simulink model "unicycle_control"  (R2015a)
settings: Solver=ode45  StartTime=0.0  StopTime=10.0  RelTol=1e-3
settings Model: Creator=Andre Coelho  LastModifiedBy=Andre Coelho

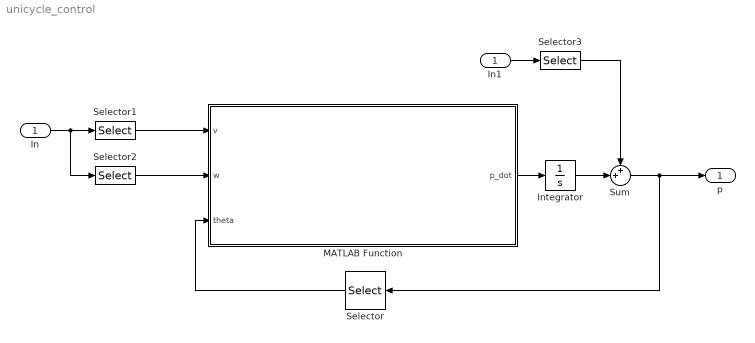
== system unicycle_control ==
  In1 : Inport
  In : InportShadow
  Integrator : Integrator  InitialCondition=[0 0 0]
  MATLAB Function : MATLAB Function  TreatAsAtomicUnit=on
  Selector : Selector  InputPortWidth=3  Indices=[3]
  Selector1 : Selector  InputPortWidth=5  Indices=[1]
  Selector2 : Selector  InputPortWidth=5  Indices=[2]
  Selector3 : Selector  InputPortWidth=5  Indices=[3:5]
  Sum : Sum  Inputs=++|
  p : Outport
  wires:
  MATLAB Function/1(p_dot) -> Integrator/1
  Selector/1 -> MATLAB Function/3(theta)
  In/1 -> Selector2/1, Selector1/1
  Integrator/1 -> Sum/2
  In1/1 -> Selector3/1
  Selector3/1 -> Sum/1
  Selector1/1 -> MATLAB Function/1(v)
  Sum/1 -> p/1, Selector/1
  Selector2/1 -> MATLAB Function/2(w)

== matlab function unicycle_control/MATLAB Function ==
  data: v input; p_dot output; w input; theta input
function p_dot = unicycle(v,w,theta)
R=1;
x_dot=v*R*cos(theta);
y_dot=v*R*sin(theta);
theta_dot=w;
p_dot=[x_dot;y_dot;theta_dot];
